simulink model "discreteFunction"  (R2023b)
settings: Solver=ode4  StartTime=0.0  StopTime=80  FixedStep=0.0833  RelTol=1e-3
settings Model: Creator=andre  LastModifiedBy=diogo
settings SolverCC: AlgebraicLoopSolver=TrustRegion
settings OptimizationCC: ReuseModelBlockBuffer=off
settings DebuggingCC: UnconnectedInputMsg=warning  UnconnectedOutputMsg=warning  UnconnectedLineMsg=warning
settings ModelReferenceCC: EnableRefExpFcnMdlSchedulingChecks=on

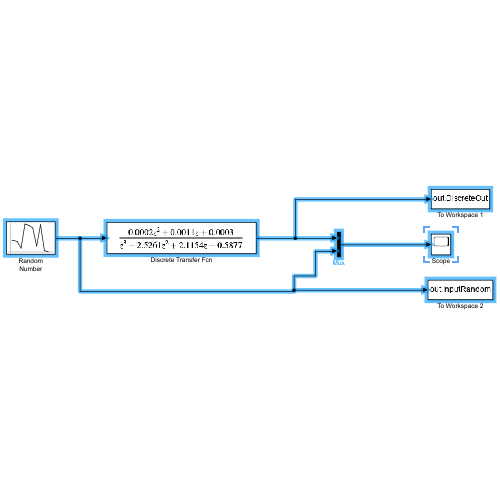
[thumbnail: Simulink's stored preview of the top-level diagram]
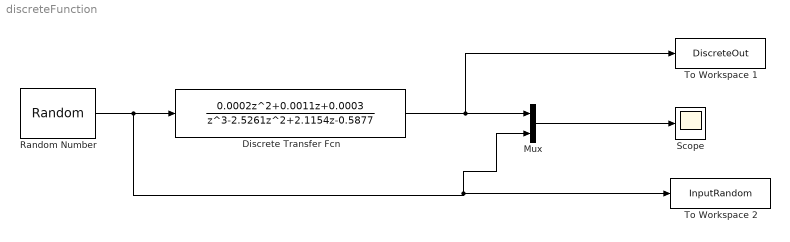
== system discreteFunction ==
  Discrete Transfer Fcn : DiscreteTransferFcn  Numerator=[0 0.0002 0.0011 0.0003]  Denominator=[1 -2.5261 2.1154 -0.5877]
  Mux : Mux  Inputs=2
  Random Number : RandomNumber  SampleTime=0.0833
  Scope : Scope
  To Workspace 1 : ToWorkspace  VariableName=DiscreteOut  SaveFormat=Timeseries  SampleTime=-1
  To Workspace 2 : ToWorkspace  VariableName=InputRandom  SaveFormat=Timeseries  SampleTime=-1
  wires:
  Random Number/1 -> Discrete Transfer Fcn/1, To Workspace 2/1, Mux/2
  Discrete Transfer Fcn/1 -> To Workspace 1/1, Mux/1
  Mux/1 -> Scope/1
